simulink model "Loops3"  (Simulink 6.0)
settings: Solver=ode45  StartTime=0.0  StopTime=10.0  RelTol=1e-3
settings Model: Creator=scaife  LastModifiedBy=scaife  ExtModeAutoUpdateStatusClock=off
settings DataIOCC: SignalLoggingName=sigsOut
settings DebuggingCC: SolverPrmCheckMsg=none
settings HardwareCC: TargetUnknown=on
settings STFCustomTargetCC: TargetFcnLib=ansi_tfl_tmw.mat  GenFloatMathFcnCalls=ANSI_C  ModelReferenceCompliant=off  SystemTargetFile=grt.tlc

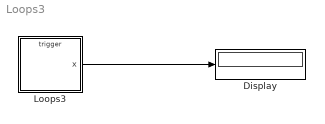
== system Loops3 ==
  Display : Display
  Loops3 : Stateflow chart
  wires:
  Loops3/1(x) -> Display/1

== stateflow chart Loops3 ==
  state A
  state B
  A -> (junction 5) : {x=0}
  (junction 6) -> B : [x>=10]
  (default) -> A
  (junction 5) -> (junction 6) : [x<10]{x++}
  (junction 6) -> (junction 5) : [x<10]{x++}
  (junction 5) -> B : [x>=10]
  B -> A
  data: x output int32
  events: event input EITHER_EDGE_EVENT
